simulink model "TESTENV_NAVI"  (R2020b)
settings: Solver=ode1  StartTime=tspan(1)  StopTime=tspan(2)  FixedStep=1/sensorFs.imuUpdateFs  RelTol=1e-3
values from neighbouring files (symbols this model uses):
  mag1 = double([Sensors.mag1.mag_x, Sensors.mag1.mag_y, Sensors.mag1.mag_z])    [navi_marg22.m]    (also in navi_marg24.m; navi_mvo17.m)
  mag2 = double([Sensors.mag2.mag_x, Sensors.mag2.mag_y, Sensors.mag2.mag_z])    [navi_marg22.m]    (also in navi_marg24.m; navi_mvo17.m)
undefined symbols (not defined in the file or in its folder): accel_x, accel_y, accel_z, ENUM_FlightTaskMode, flightControlMode, flightTaskMode, IMU1, IMU2, IMU3, mag_x, mag_y, mag_z, PlaneMode, SIM_SENSOR_SET, uavMode, VISLANDING_PARAM_V10, VISLANDING_PARAM_V1000
settings Model: PauseTimes=266.88  Creator=sl  LastModifiedBy=sl
settings SolverCC: AutoInsertRateTranBlk=on
settings OptimizationCC: DefaultParameterBehavior=Inlined  EnhancedBackFolding=on  PassReuseOutputArgsAs=Individual arguments  ZeroExternalMemoryAtStartup=off  ZeroInternalMemoryAtStartup=off  MaxStackSize=64  OptimizeBlockOrder=speed  DifferentSizesBufferReuse=on  OptimizationCustomize=off  EfficientTunableParamExpr=on
settings DebuggingCC: MultiTaskCondExecSysMsg=none  ParameterPrecisionLossMsg=none  ParameterTunabilityLossMsg=error  UnconnectedInputMsg=none  UnconnectedOutputMsg=none  UnconnectedLineMsg=none  BusObjectLabelMismatch=error
settings HardwareCC: ProdBitPerPointer=32  ProdBitPerSizeT=32  ProdBitPerPtrDiffT=32  ProdLargestAtomicInteger=Long  ProdLargestAtomicFloat=Double  ProdWordSize=32  ProdHWDeviceType=ARM Compatible->ARM Cortex
settings ModelReferenceCC: EnableParallelModelReferenceBuilds=on  ParallelModelReferenceMATLABWorkerInit=Load Top Model
settings SFSimCC: MATLABDynamicMemAlloc=off
settings RTWCC: Description=Embedded Coder  SystemTargetFile=ert.tlc  TemplateMakefile=ert_default_tmf  GenerateReport=on  Toolchain=GNU Tools for ARM Embedded Processors  IncludeHyperlinkInReport=on  LaunchReport=on  GenerateTraceInfo=on  GenerateTraceReport=on  GenerateTraceReportSl=on  GenerateTraceReportSf=on  GenerateTraceReportEml=on
settings CodeAppCC: ForceParamTrailComments=on  IgnoreCustomStorageClasses=off  OperatorAnnotations=on  SimulinkDataObjDesc=on  SFDataObjDesc=on  InsertBlockDesc=on
settings ERTTargetCC: InlinedParameterPlacement=NonHierarchical  ERTCustomFileTemplate=example_file_process.tlc

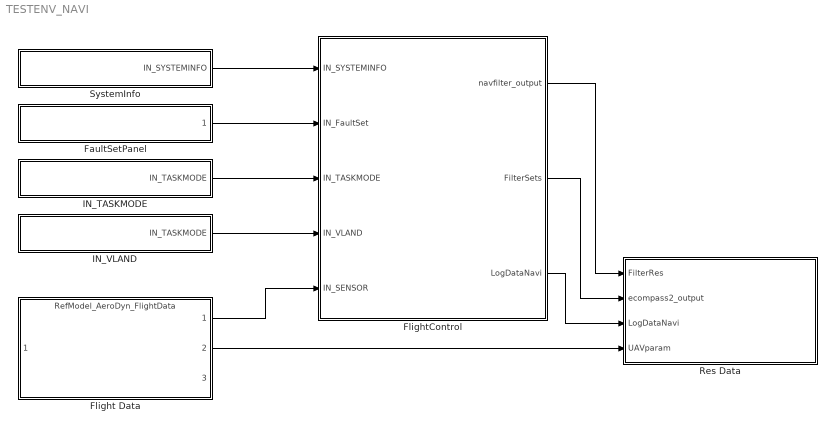
== system TESTENV_NAVI ==
  FaultSetPanel : ModelReference  ModelNameDialog=RefModel_FaultPanel  SimulationMode=Normal  ModelReferenceVersion=2.3
  Flight Data : ModelReference  DisableCoverage=on  ModelNameDialog=RefModel_AeroDyn_FlightData.slx  SimulationMode=Normal  ModelReferenceVersion=2.45
  FlightControl : Subsystem
  IN_TASKMODE : Subsystem
  IN_VLAND : Subsystem
  Res Data : Subsystem  VariantControl=SimulinkRunMode == 1
  SystemInfo : Subsystem
  wires:
  FlightControl/1(navfilter_output) -> Res Data/1(FilterRes)
  FlightControl/2(FilterSets) -> Res Data/2(ecompass2_output)
  Flight Data/1 -> FlightControl/5(IN_SENSOR)
  Flight Data/2 -> Res Data/4(UAVparam)
  FaultSetPanel/1 -> FlightControl/2(IN_FaultSet)
  SystemInfo/1(IN_SYSTEMINFO) -> FlightControl/1(IN_SYSTEMINFO)
  IN_TASKMODE/1(IN_TASKMODE) -> FlightControl/3(IN_TASKMODE)
  IN_VLAND/1(IN_TASKMODE) -> FlightControl/4(IN_VLAND)
  FlightControl/3(LogDataNavi) -> Res Data/3(LogDataNavi)

== system TESTENV_NAVI/FlightControl ==
  IN_SYSTEMINFO : Inport
  IN_FaultSet : Inport  Port=2
  IN_TASKMODE : Inport  Port=3
  IN_VLAND : Inport  Port=4
  IN_SENSOR : Inport  Port=5
  Bus Selector : BusSelector  OutputSignals=OUT_NaviFilter.Status.initialAlignmentComplete
  SensorAndNavigation1 : Subsystem
  TEST_Filter : Subsystem
  navfilter_output : Outport
  FilterSets : Outport  Port=2
  LogDataNavi : Outport  Port=3
  wires:
  SensorAndNavigation1/1(OUT_Navi) -> Bus Selector/1, navfilter_output/1
  IN_SENSOR/1 -> SensorAndNavigation1/1(IN_Sensor), TEST_Filter/1(In1)
  IN_FaultSet/1 -> SensorAndNavigation1/2(IN_FaultSet)
  TEST_Filter/1(Out1) -> FilterSets/1
  IN_SYSTEMINFO/1 -> SensorAndNavigation1/3(IN_SystemInfo)
  IN_TASKMODE/1 -> SensorAndNavigation1/4(IN_TASKMODE)
  IN_VLAND/1 -> SensorAndNavigation1/5(IN_VLandmark)
  SensorAndNavigation1/4(LogDataNavi) -> LogDataNavi/1

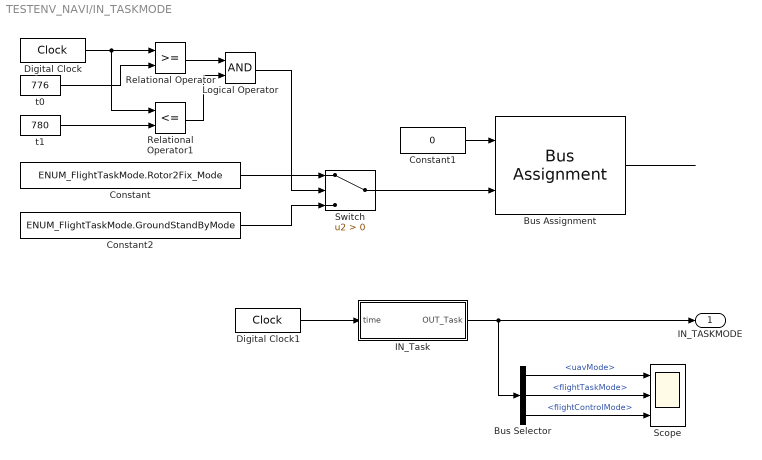
== system TESTENV_NAVI/IN_TASKMODE ==
  Bus Assignment : BusAssignment  AssignedSignals=flightTaskMode
  Bus Selector : BusSelector  OutputSignals=uavMode,flightTaskMode,flightControlMode
  Constant : Constant  Value=ENUM_FlightTaskMode.Rotor2Fix_Mode  OutDataTypeStr=Enum: ENUM_FlightTaskMode
  Constant1 : Constant  Value=0  OutDataTypeStr=Bus: BUS_TASK_PATH_OutParam
  Constant2 : Constant  Value=ENUM_FlightTaskMode.GroundStandByMode  OutDataTypeStr=Enum: ENUM_FlightTaskMode
  Digital Clock : DigitalClock  SampleTime=-1
  Digital Clock1 : DigitalClock  SampleTime=-1
  IN_Task : Subsystem
  Logical Operator : Logic  AllPortsSameDT=off  OutDataTypeStr=boolean
  Relational Operator : RelationalOperator  OutDataTypeStr=boolean  RndMeth=Simplest
  Relational Operator1 : RelationalOperator  Operator=<=  OutDataTypeStr=boolean  RndMeth=Simplest
  Scope : Scope  NumInputPorts=3
  Switch : Switch  Criteria=u2 > Threshold
  t0 : Constant  Value=776
  t1 : Constant  Value=780
  IN_TASKMODE : Outport
  wires:
  Bus Assignment/1 -> ?
  Constant/1 -> Switch/1
  Constant1/1 -> Bus Assignment/1
  Switch/1 -> Bus Assignment/2
  Constant2/1 -> Switch/3
  Logical Operator/1 -> Switch/2
  Digital Clock/1 -> Relational Operator1/1, Relational Operator/1
  t0/1 -> Relational Operator/2
  t1/1 -> Relational Operator1/2
  Relational Operator/1 -> Logical Operator/1
  Relational Operator1/1 -> Logical Operator/2
  Digital Clock1/1 -> IN_Task/1(time)
  IN_Task/1(OUT_Task) -> Bus Selector/1, IN_TASKMODE/1
  Bus Selector/1 -> Scope/1  "<uavMode>"
  Bus Selector/2 -> Scope/2  "<flightTaskMode>"
  Bus Selector/3 -> Scope/3  "<flightControlMode>"

== system TESTENV_NAVI/IN_VLAND ==
  Bus Assignment : BusAssignment  AssignedSignals=time
  Constant1 : Constant  Value=0  OutDataTypeStr=Bus: BUS_VISUALLANDING_INPUT
  IN_TASKMODE : Outport
  wires:
  Constant1/1 -> Bus Assignment/1
  Bus Assignment/1 -> IN_TASKMODE/1

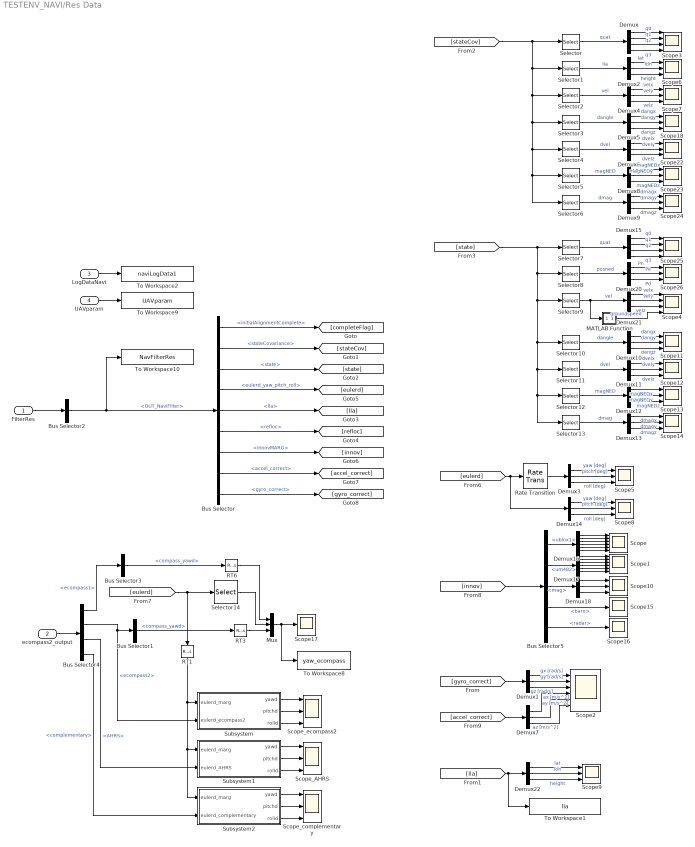
== system TESTENV_NAVI/Res Data ==
  FilterRes : Inport
  ecompass2_output : Inport  Port=2
  LogDataNavi : Inport  Port=3
  UAVparam : Inport  Port=4
  Bus Selector : BusSelector  OutputSignals=Status.initialAlignmentComplete,stateCovariance,state,eulerd_yaw_pitch_roll,lla,InitValue.refloc,innovMARG,accel_correct,gyro_correct
  Bus Selector1 : BusSelector  OutputSignals=compass_yawd
  Bus Selector2 : BusSelector  OutputSignals=OUT_NaviFilter
  Bus Selector3 : BusSelector  OutputSignals=compass_yawd
  Bus Selector4 : BusSelector  OutputSignals=ecompass1,ecompass2,AHRS,complementary
  Bus Selector5 : BusSelector  OutputSignals=ublox1,um482,mag,baro,radar
  Demux : Demux
  Demux{1..14,18,20..22} (18 alike) : Demux  Outputs=3
  Demux15 : Demux
  Demux16 : Demux  Outputs=6
  Demux17 : Demux  Outputs=6
  MATLAB Function : MATLAB Function  TreatAsAtomicUnit=on
  Mux : Mux  Inputs=3
  RT1 : RateTransition
  RT3 : RateTransition
  RT6 : RateTransition
  Rate Transition : RateTransition
  Scope : Scope  NumInputPorts=6
  Scope1 : Scope  NumInputPorts=6
  Scope{5..14,18,22..24,26} (15 alike) : Scope  NumInputPorts=3
  Scope15 : Scope
  Scope16 : Scope
  Scope17 : Scope
  Scope2 : Scope  NumInputPorts=6
  Scope25 : Scope  NumInputPorts=4
  Scope3 : Scope  NumInputPorts=4
  Scope4 : Scope  NumInputPorts=4
  Scope_AHRS : Scope  NumInputPorts=3
  Scope_complementary : Scope  NumInputPorts=3
  Scope_ecompass2 : Scope  NumInputPorts=3
  Selector : Selector  InputPortWidth=nStateMARG24  IndexOptions=Index vector (dialog)  Indices=[1:4]  OutputSizes=1
  Selector1 : Selector  InputPortWidth=nStateMARG24  IndexOptions=Index vector (dialog)  Indices=[5:7]  OutputSizes=1
  Selector10 : Selector  InputPortWidth=nStateMARG24  IndexOptions=Index vector (dialog)  Indices=[11:13]  OutputSizes=1
  Selector11 : Selector  InputPortWidth=nStateMARG24  IndexOptions=Index vector (dialog)  Indices=[14:16]  OutputSizes=1
  Selector12 : Selector  InputPortWidth=nStateMARG24  IndexOptions=Index vector (dialog)  Indices=[17:19]  OutputSizes=1
  Selector13 : Selector  InputPortWidth=nStateMARG24  IndexOptions=Index vector (dialog)  Indices=[20:22]  OutputSizes=1
  Selector14 : Selector  InputPortWidth=3  IndexOptions=Index vector (dialog)  Indices=1  OutputSizes=1
  Selector2 : Selector  InputPortWidth=nStateMARG24  IndexOptions=Index vector (dialog)  Indices=[8:10]  OutputSizes=1
  Selector3 : Selector  InputPortWidth=nStateMARG24  IndexOptions=Index vector (dialog)  Indices=[11:13]  OutputSizes=1
  Selector4 : Selector  InputPortWidth=nStateMARG24  IndexOptions=Index vector (dialog)  Indices=[14:16]  OutputSizes=1
  Selector5 : Selector  InputPortWidth=nStateMARG24  IndexOptions=Index vector (dialog)  Indices=[17:19]  OutputSizes=1
  Selector6 : Selector  InputPortWidth=nStateMARG24  IndexOptions=Index vector (dialog)  Indices=[20:22]  OutputSizes=1
  Selector7 : Selector  InputPortWidth=nStateMARG24  IndexOptions=Index vector (dialog)  Indices=[1:4]  OutputSizes=1
  Selector8 : Selector  InputPortWidth=nStateMARG24  IndexOptions=Index vector (dialog)  Indices=[5:7]  OutputSizes=1
  Selector9 : Selector  InputPortWidth=nStateMARG24  IndexOptions=Index vector (dialog)  Indices=[8:10]  OutputSizes=1
  Subsystem : Subsystem
  Subsystem1 : Subsystem
  Subsystem2 : Subsystem
  To Workspace1 : ToWorkspace  VariableName=lla  SaveFormat=Timeseries  SampleTime=-1
  To Workspace10 : ToWorkspace  VariableName=NavFilterRes  SaveFormat=Timeseries  SampleTime=-1
  To Workspace2 : ToWorkspace  VariableName=naviLogData1  SaveFormat=Timeseries  SampleTime=-1
  To Workspace8 : ToWorkspace  VariableName=yaw_ecompass  SaveFormat=Timeseries  SampleTime=-1
  To Workspace9 : ToWorkspace  VariableName=UAVparam  SaveFormat=Timeseries  SampleTime=-1
  wires:
  Demux13/1 -> Scope14/1  "dmagx"
  Demux21/3 -> Scope4/3  "velz"
  Demux12/1 -> Scope13/1  "magNEDx"
  Selector14/1 -> Mux/2
  Demux10/1 -> Scope11/1  "dangx"
  Demux12/2 -> Scope13/2  "magNEDy"
  Selector10/1 -> Demux10/1  "dangle"
  Demux15/4 -> Scope25/4  "q3"
  Selector1/1 -> Demux2/1  "lla"
  Demux3/2 -> Scope5/2  "pitch [deg]"
  [state] -> Selector8/1, Selector11/1, Selector12/1, Selector13/1, Selector10/1, Selector9/1, Selector7/1
  Demux5/2 -> Scope18/2  "dangy"
  Selector12/1 -> Demux12/1  "magNED"
  Selector13/1 -> Demux13/1  "dmag"
  Demux11/1 -> Scope12/1  "dvelx"
  [innov] -> Bus Selector5/1
  Demux11/2 -> Scope12/2  "dvely"
  Demux15/3 -> Scope25/3  "q2"
  Demux6/3 -> Scope22/3  "dvelz"
  Mux/1 -> To Workspace8/1, Scope17/1
  Demux15/2 -> Scope25/2  "q1"
  Bus Selector1/1 -> RT3/1  "<compass_yawd>"
  [eulerd] -> Demux14/1, Rate Transition/1
  [eulerd] -> Selector14/1, RT1/1
  Demux10/3 -> Scope11/3  "dangz"
  Demux21/1 -> Scope4/1  "velx"
  Demux/2 -> Scope3/2  "q1"
  Demux/1 -> Scope3/1  "q0"
  [stateCov] -> Selector/1, Selector3/1, Selector4/1, Selector5/1, Selector6/1, Selector2/1, Selector1/1
  Demux9/2 -> Scope24/2  "dmagy"
  Demux/3 -> Scope3/3  "q2"
  Selector2/1 -> Demux4/1  "vel"
  Demux13/2 -> Scope14/2  "dmagy"
  Selector6/1 -> Demux9/1  "dmag"
  RT3/1 -> Mux/3
  Demux/4 -> Scope3/4  "q3"
  Demux2/1 -> Scope6/1  "lat"
  Demux2/3 -> Scope6/3  "height"
  Selector/1 -> Demux/1  "quat"
  Demux5/3 -> Scope18/3  "dangz"
  Demux4/3 -> Scope7/3  "velz"
  Demux10/2 -> Scope11/2  "dangy"
  Demux4/2 -> Scope7/2  "vely"
  Demux8/2 -> Scope23/2  "magNEDy"
  Selector3/1 -> Demux5/1  "dangle"
  Demux2/2 -> Scope6/2  "lon"
  Selector5/1 -> Demux8/1  "magNED"
  Demux8/1 -> Scope23/1  "magNEDx"
  Demux6/2 -> Scope22/2  "dvely"
  Demux9/3 -> Scope24/3  "dmagz"
  Demux12/3 -> Scope13/3  "magNEDz"
  Demux3/3 -> Scope5/3  "roll [deg]"
  Demux21/2 -> Scope4/2  "vely"
  Demux8/3 -> Scope23/3  "magNEDz"
  Selector11/1 -> Demux11/1  "dvel"
  Selector9/1 -> MATLAB Function/1(vel), Demux21/1  "vel"
  Demux20/3 -> Scope26/3  "Pd"
  Selector7/1 -> Demux15/1  "quat"
  Demux13/3 -> Scope14/3  "dmagz"
  Demux20/2 -> Scope26/2  "Pe"
  Selector4/1 -> Demux6/1  "dvel"
  Selector8/1 -> Demux20/1  "posned"
  Demux3/1 -> Scope5/1  "yaw [deg]"
  Demux11/3 -> Scope12/3  "dvelz"
  Demux15/1 -> Scope25/1  "q0"
  Demux20/1 -> Scope26/1  "Pn"
  Demux5/1 -> Scope18/1  "dangx"
  Demux6/1 -> Scope22/1  "dvelx"
  Demux4/1 -> Scope7/1  "velx"
  Demux9/1 -> Scope24/1  "dmagx"
  FilterRes/1 -> Bus Selector2/1
  Bus Selector/4 -> [eulerd]  "<eulerd_yaw_pitch_roll>"
  Bus Selector/3 -> [state]  "<state>"
  Bus Selector/5 -> [lla]  "<lla>"
  Bus Selector/2 -> [stateCov]  "<stateCovariance>"
  Bus Selector/6 -> [refloc]  "<refloc>"
  Bus Selector/1 -> [completeFlag]  "<initialAlignmentComplete>"
  Bus Selector/7 -> [innov]  "<innovMARG>"
  ecompass2_output/1 -> Bus Selector4/1
  Bus Selector/8 -> [accel_correct]  "<accel_correct>"
  Bus Selector/9 -> [gyro_correct]  "<gyro_correct>"
  [gyro_correct] -> Demux1/1
  [accel_correct] -> Demux7/1
  Demux1/1 -> Scope2/1  "gx [rad/s]"
  Demux1/2 -> Scope2/2  "gy [rad/s]"
  Demux1/3 -> Scope2/3  "gz [rad/s]"
  Demux7/1 -> Scope2/4  "ax [m/s^2]"
  Demux7/2 -> Scope2/5  "ay [m/s^2]"
  Demux7/3 -> Scope2/6  "az [m/s^2]"
  UAVparam/1 -> To Workspace9/1
  Rate Transition/1 -> Demux3/1
  Demux14/1 -> Scope8/1  "yaw [deg]"
  Demux14/3 -> Scope8/3  "roll [deg]"
  Demux14/2 -> Scope8/2  "pitch [deg]"
  Demux22/2 -> Scope9/2  "lon"
  Demux22/3 -> Scope9/3  "height"
  Demux22/1 -> Scope9/1  "lat"
  [lla] -> To Workspace1/1, Demux22/1
  Bus Selector3/1 -> RT6/1  "<compass_yawd>"
  RT6/1 -> Mux/1
  Bus Selector4/2 -> Subsystem/2(eulerd_ecompass2), Bus Selector1/1  "<ecompass2>"
  Bus Selector4/1 -> Bus Selector3/1  "<ecompass1>"
  Bus Selector4/3 -> Subsystem1/2(eulerd_AHRS)  "<AHRS>"
  RT1/1 -> Subsystem2/1(eulerd_marg), Subsystem1/1(eulerd_marg), Subsystem/1(eulerd_marg)
  Subsystem/1(yawd) -> Scope_ecompass2/1
  Subsystem/2(pitchd) -> Scope_ecompass2/2
  Subsystem/3(rolld) -> Scope_ecompass2/3
  Subsystem1/3(rolld) -> Scope_AHRS/3
  Subsystem1/2(pitchd) -> Scope_AHRS/2
  Subsystem1/1(yawd) -> Scope_AHRS/1
  Subsystem2/1(yawd) -> Scope_complementary/1
  Subsystem2/2(pitchd) -> Scope_complementary/2
  Subsystem2/3(rolld) -> Scope_complementary/3
  Bus Selector4/4 -> Subsystem2/2(eulerd_complementary)  "<complementary>"
  MATLAB Function/1(y) -> Scope4/4  "groundspeed"
  Bus Selector2/1 -> To Workspace10/1, Bus Selector/1  "<OUT_NaviFilter>"
  LogDataNavi/1 -> To Workspace2/1
  Bus Selector5/1 -> Demux16/1  "<ublox1>"
  Demux16/1 -> Scope/1
  Demux16/2 -> Scope/2
  Demux16/3 -> Scope/3
  Demux16/4 -> Scope/4
  Demux16/5 -> Scope/5
  Demux16/6 -> Scope/6
  Demux17/6 -> Scope1/6
  Demux17/5 -> Scope1/5
  Demux17/4 -> Scope1/4
  Demux17/3 -> Scope1/3
  Demux17/2 -> Scope1/2
  Demux17/1 -> Scope1/1
  Bus Selector5/2 -> Demux17/1  "<um482>"
  Bus Selector5/3 -> Demux18/1  "<mag>"
  Demux18/1 -> Scope10/1
  Demux18/2 -> Scope10/2
  Demux18/3 -> Scope10/3
  Bus Selector5/4 -> Scope15/1  "<baro>"
  Bus Selector5/5 -> Scope16/1  "<radar>"

== system TESTENV_NAVI/SystemInfo ==
  Bus Assignment : BusAssignment  AssignedSignals=plane_model_control
  Constant : Constant  Value=PlaneMode.mode  OutDataTypeStr=Enum: ENUM_plane_mode
  Constant1 : Constant  Value=0  OutDataTypeStr=Bus: BUS_SYSTEMINFO_INPUT
  IN_SYSTEMINFO : Outport
  wires:
  Constant1/1 -> Bus Assignment/1
  Constant/1 -> Bus Assignment/2
  Bus Assignment/1 -> IN_SYSTEMINFO/1

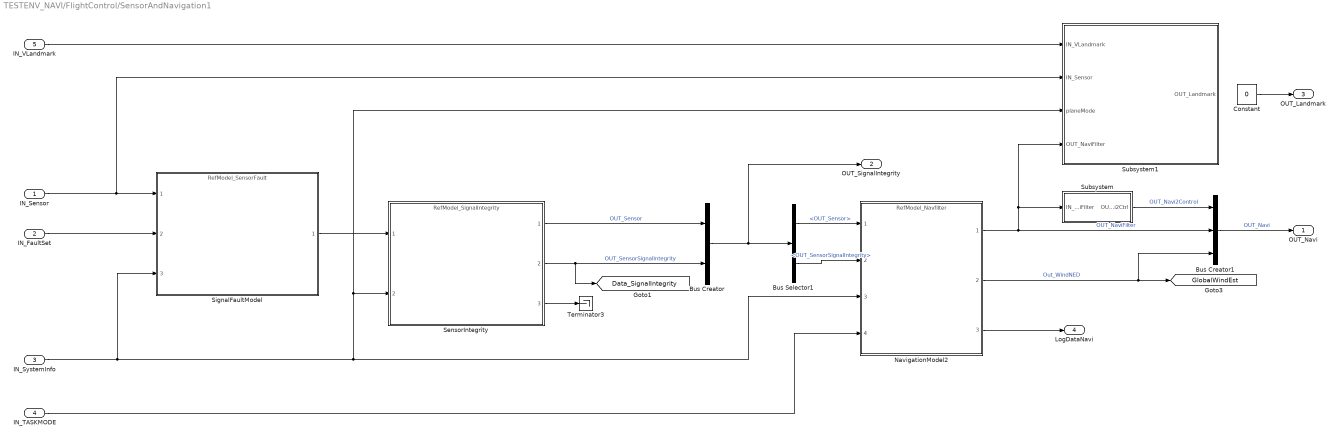
== system TESTENV_NAVI/FlightControl/SensorAndNavigation1 ==
  IN_Sensor : Inport
  IN_FaultSet : Inport  Port=2
  IN_SystemInfo : Inport  Port=3
  IN_TASKMODE : Inport  Port=4
  IN_VLandmark : Inport  Port=5
  Bus Creator : BusCreator  Inputs=2
  Bus Creator1 : BusCreator  Inputs=3
  Bus Selector1 : BusSelector  OutputSignals=OUT_Sensor,OUT_SensorSignalIntegrity
  Constant : Constant  Value=0  OutDataTypeStr=Bus: BUS_VISUALLANDING_LANDMARK
  NavigationModel2 : ModelReference  ModelNameDialog=RefModel_Navfilter  SimulationMode=Normal  CachedPortDiscreteRates=[0.004]  ModelReferenceVersion=2.1363
  SensorIntegrity : ModelReference  ModelNameDialog=RefModel_SignalIntegrity  SimulationMode=Normal  CachedPortDiscreteRates=[0.004]  ModelReferenceVersion=2.46
  SignalFaultModel : ModelReference  DisableCoverage=on  ModelNameDialog=RefModel_SensorFault.slx  SimulationMode=Normal  ModelReferenceVersion=2.1
  Subsystem : Subsystem
  Subsystem1 : Subsystem
  Terminator3 : Terminator
  OUT_Navi : Outport
  OUT_SignalIntegrity : Outport  Port=2
  OUT_Landmark : Outport  Port=3  OutDataTypeStr=Bus: BUS_VISUALLANDING_LANDMARK
  LogDataNavi : Outport  Port=4
  tag scope: Data_SignalIntegrity=global, GlobalWindEst=global
  wires:
  Bus Creator1/1 -> OUT_Navi/1  "OUT_Navi"
  IN_FaultSet/1 -> SignalFaultModel/2
  IN_Sensor/1 -> Subsystem1/2(IN_Sensor), SignalFaultModel/1
  SensorIntegrity/3 -> Terminator3/1
  SensorIntegrity/1 -> Bus Creator/1  "OUT_Sensor"
  SensorIntegrity/2 -> [Data_SignalIntegrity], Bus Creator/2  "OUT_SensorSignalIntegrity"
  SignalFaultModel/1 -> SensorIntegrity/1
  Subsystem/1(OUT_Navi2Ctrl) -> Bus Creator1/1  "OUT_Navi2Control"
  NavigationModel2/2 -> [GlobalWindEst], Bus Creator1/3  "Out_WindNED"
  Bus Creator/1 -> Bus Selector1/1, OUT_SignalIntegrity/1
  Bus Selector1/2 -> NavigationModel2/2  "<OUT_SensorSignalIntegrity>"
  Bus Selector1/1 -> NavigationModel2/1  "<OUT_Sensor>"
  NavigationModel2/1 -> Subsystem/1(IN_NaviFilter), Subsystem1/4(OUT_NaviFilter), Bus Creator1/2  "OUT_NaviFilter"
  IN_SystemInfo/1 -> Subsystem1/3(planeMode), SensorIntegrity/2, NavigationModel2/3, SignalFaultModel/3
  IN_TASKMODE/1 -> NavigationModel2/4
  IN_VLandmark/1 -> Subsystem1/1(IN_VLandmark)
  NavigationModel2/3 -> LogDataNavi/1
  Constant/1 -> OUT_Landmark/1

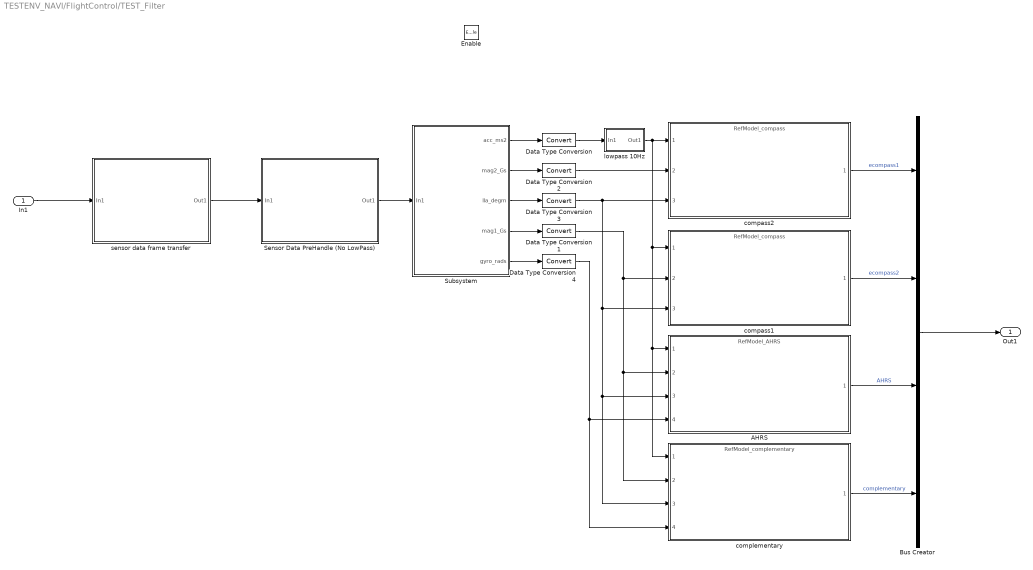
== system TESTENV_NAVI/FlightControl/TEST_Filter ==
  In1 : Inport
  Enable : EnablePort
  AHRS : ModelReference  ModelNameDialog=RefModel_AHRS.slx  SimulationMode=Normal  ModelReferenceVersion=2.3
  Bus Creator : BusCreator  Inputs=4
  Data Type Conversion{,1..4} (5 alike) : DataTypeConversion
  Sensor Data PreHandle (No LowPass) : Subsystem
  Subsystem : Subsystem
  compass1 : ModelReference  ModelNameDialog=RefModel_compass.slx  SimulationMode=Normal  ModelReferenceVersion=2.0
  compass2 : ModelReference  ModelNameDialog=RefModel_compass.slx  SimulationMode=Normal  ModelReferenceVersion=2.0
  complementary : ModelReference  ModelNameDialog=RefModel_complementary.slx  SimulationMode=Normal  ModelReferenceVersion=2.0
  lowpass 10Hz : Subsystem
  sensor data frame transfer : Subsystem
  Out1 : Outport
  wires:
  Sensor Data PreHandle (No LowPass)/1(Out1) -> Subsystem/1(In1)
  sensor data frame transfer/1(Out1) -> Sensor Data PreHandle (No LowPass)/1(In1)
  Data Type Conversion/1 -> lowpass 10Hz/1(In1)
  Subsystem/1(acc_ms2) -> Data Type Conversion/1
  Subsystem/2(mag2_Gs) -> Data Type Conversion2/1
  Data Type Conversion2/1 -> compass2/2
  lowpass 10Hz/1(Out1) -> complementary/1, AHRS/1, compass1/1, compass2/1
  Subsystem/4(mag1_Gs) -> Data Type Conversion1/1
  Data Type Conversion4/1 -> complementary/4, AHRS/4
  Data Type Conversion3/1 -> complementary/3, AHRS/3, compass1/3, compass2/3
  Data Type Conversion1/1 -> complementary/2, AHRS/2, compass1/2
  Subsystem/3(lla_degm) -> Data Type Conversion3/1
  Subsystem/5(gyro_rads) -> Data Type Conversion4/1
  AHRS/1 -> Bus Creator/3  "AHRS"
  complementary/1 -> Bus Creator/4  "complementary"
  Bus Creator/1 -> Out1/1
  compass2/1 -> Bus Creator/1  "ecompass1"
  compass1/1 -> Bus Creator/2  "ecompass2"
  In1/1 -> sensor data frame transfer/1(In1)

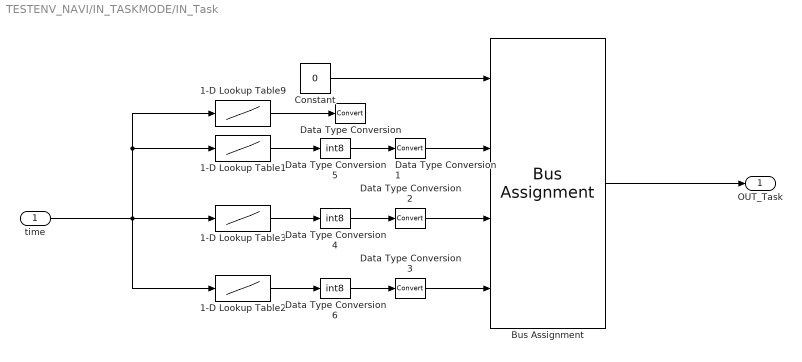
== system TESTENV_NAVI/IN_TASKMODE/IN_Task ==
  time : Inport
  1-D Lookup Table1 : Lookup_n-D  NumberOfTableDimensions=1  BreakpointsForDimension1=IN_Task.time_cal(1:end-20)  Table=IN_Task.uavMode(1:end-20)  InterpMethod=Flat  ExtrapMethod=Clip  InternalRulePriority=Speed  RndMeth=Simplest  InputSameDT=on
  1-D Lookup Table2 : Lookup_n-D  NumberOfTableDimensions=1  BreakpointsForDimension1=IN_Task.time_cal(1:end-20)  Table=IN_Task.flightControlMode(1:end-20)  InterpMethod=Flat  ExtrapMethod=Clip  InternalRulePriority=Speed  RndMeth=Simplest  InputSameDT=on
  1-D Lookup Table3 : Lookup_n-D  NumberOfTableDimensions=1  BreakpointsForDimension1=IN_Task.time_cal(1:end-20)  Table=IN_Task.flightTaskMode(1:end-20)  InterpMethod=Flat  ExtrapMethod=Clip  InternalRulePriority=Speed  RndMeth=Simplest  InputSameDT=on
  1-D Lookup Table9 : Lookup_n-D  NumberOfTableDimensions=1  BreakpointsForDimension1=IN_Task.time_cal(1:end-20)  Table=IN_Task.time_cal(1:end-20)  InterpMethod=Flat  ExtrapMethod=Clip  InternalRulePriority=Speed  RndMeth=Simplest  InputSameDT=on
  Bus Assignment : BusAssignment  AssignedSignals=uavMode,flightTaskMode,flightControlMode
  Constant : Constant  Value=0  OutDataTypeStr=Bus: BUS_TASK_PATH_OutParam
  Data Type Conversion{,1..3} (4 alike) : DataTypeConversion
  Data Type Conversion4 : DataTypeConversion  OutDataTypeStr=int8
  Data Type Conversion5 : DataTypeConversion  OutDataTypeStr=int8
  Data Type Conversion6 : DataTypeConversion  OutDataTypeStr=int8
  OUT_Task : Outport
  wires:
  Bus Assignment/1 -> OUT_Task/1
  1-D Lookup Table9/1 -> Data Type Conversion/1
  1-D Lookup Table1/1 -> Data Type Conversion5/1
  1-D Lookup Table3/1 -> Data Type Conversion4/1
  1-D Lookup Table2/1 -> Data Type Conversion6/1
  time/1 -> 1-D Lookup Table2/1, 1-D Lookup Table3/1, 1-D Lookup Table1/1, 1-D Lookup Table9/1
  Constant/1 -> Bus Assignment/1
  Data Type Conversion1/1 -> Bus Assignment/2
  Data Type Conversion2/1 -> Bus Assignment/3
  Data Type Conversion3/1 -> Bus Assignment/4
  Data Type Conversion6/1 -> Data Type Conversion3/1
  Data Type Conversion5/1 -> Data Type Conversion1/1
  Data Type Conversion4/1 -> Data Type Conversion2/1

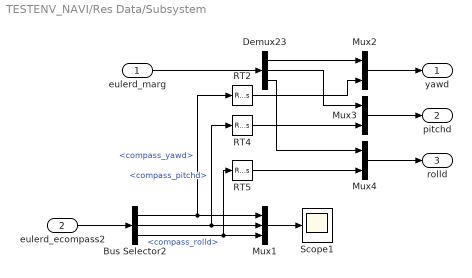
== system TESTENV_NAVI/Res Data/Subsystem ==
  eulerd_marg : Inport
  eulerd_ecompass2 : Inport  Port=2
  Bus Selector2 : BusSelector  OutputSignals=compass_yawd,compass_pitchd,compass_rolld
  Demux23 : Demux  Outputs=3
  Mux1 : Mux  Inputs=3
  Mux2 : Mux  Inputs=2
  Mux3 : Mux  Inputs=2
  Mux4 : Mux  Inputs=2
  RT2 : RateTransition
  RT4 : RateTransition
  RT5 : RateTransition
  Scope1 : Scope
  yawd : Outport
  pitchd : Outport  Port=2
  rolld : Outport  Port=3
  wires:
  RT4/1 -> Mux3/2
  Demux23/1 -> Mux2/1
  RT2/1 -> Mux2/2
  Mux1/1 -> Scope1/1
  Bus Selector2/2 -> RT4/1, Mux1/2  "<compass_pitchd>"
  Demux23/3 -> Mux4/1
  eulerd_marg/1 -> Demux23/1
  Bus Selector2/3 -> RT5/1, Mux1/3  "<compass_rolld>"
  RT5/1 -> Mux4/2
  Demux23/2 -> Mux3/1
  Bus Selector2/1 -> Mux1/1, RT2/1  "<compass_yawd>"
  Mux4/1 -> rolld/1
  eulerd_ecompass2/1 -> Bus Selector2/1
  Mux3/1 -> pitchd/1
  Mux2/1 -> yawd/1

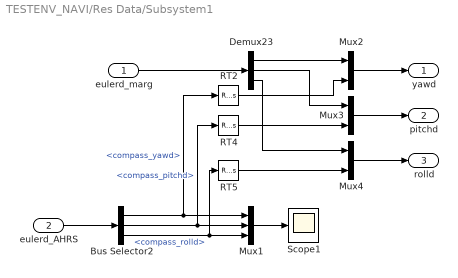
== system TESTENV_NAVI/Res Data/Subsystem1 ==
  eulerd_marg : Inport
  eulerd_AHRS : Inport  Port=2
  Bus Selector2 : BusSelector  OutputSignals=compass_yawd,compass_pitchd,compass_rolld
  Demux23 : Demux  Outputs=3
  Mux1 : Mux  Inputs=3
  Mux2 : Mux  Inputs=2
  Mux3 : Mux  Inputs=2
  Mux4 : Mux  Inputs=2
  RT2 : RateTransition
  RT4 : RateTransition
  RT5 : RateTransition
  Scope1 : Scope
  yawd : Outport
  pitchd : Outport  Port=2
  rolld : Outport  Port=3
  wires:
  Mux2/1 -> yawd/1
  Mux3/1 -> pitchd/1
  eulerd_AHRS/1 -> Bus Selector2/1
  Mux4/1 -> rolld/1
  Bus Selector2/1 -> RT2/1, Mux1/1  "<compass_yawd>"
  Demux23/2 -> Mux3/1
  RT5/1 -> Mux4/2
  Bus Selector2/3 -> Mux1/3, RT5/1  "<compass_rolld>"
  eulerd_marg/1 -> Demux23/1
  Demux23/3 -> Mux4/1
  Bus Selector2/2 -> Mux1/2, RT4/1  "<compass_pitchd>"
  Mux1/1 -> Scope1/1
  RT2/1 -> Mux2/2
  Demux23/1 -> Mux2/1
  RT4/1 -> Mux3/2

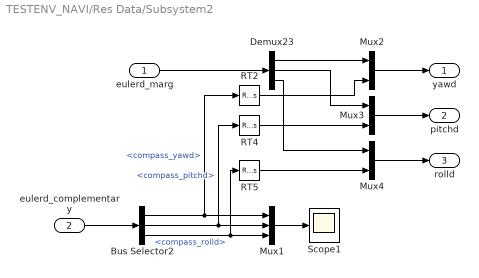
== system TESTENV_NAVI/Res Data/Subsystem2 ==
  eulerd_marg : Inport
  eulerd_complementary : Inport  Port=2
  Bus Selector2 : BusSelector  OutputSignals=compass_yawd,compass_pitchd,compass_rolld
  Demux23 : Demux  Outputs=3
  Mux1 : Mux  Inputs=3
  Mux2 : Mux  Inputs=2
  Mux3 : Mux  Inputs=2
  Mux4 : Mux  Inputs=2
  RT2 : RateTransition
  RT4 : RateTransition
  RT5 : RateTransition
  Scope1 : Scope
  yawd : Outport
  pitchd : Outport  Port=2
  rolld : Outport  Port=3
  wires:
  RT4/1 -> Mux3/2
  Demux23/1 -> Mux2/1
  RT2/1 -> Mux2/2
  Mux1/1 -> Scope1/1
  Bus Selector2/2 -> RT4/1, Mux1/2  "<compass_pitchd>"
  Demux23/3 -> Mux4/1
  eulerd_marg/1 -> Demux23/1
  Bus Selector2/3 -> RT5/1, Mux1/3  "<compass_rolld>"
  RT5/1 -> Mux4/2
  Demux23/2 -> Mux3/1
  Bus Selector2/1 -> Mux1/1, RT2/1  "<compass_yawd>"
  Mux4/1 -> rolld/1
  eulerd_complementary/1 -> Bus Selector2/1
  Mux3/1 -> pitchd/1
  Mux2/1 -> yawd/1

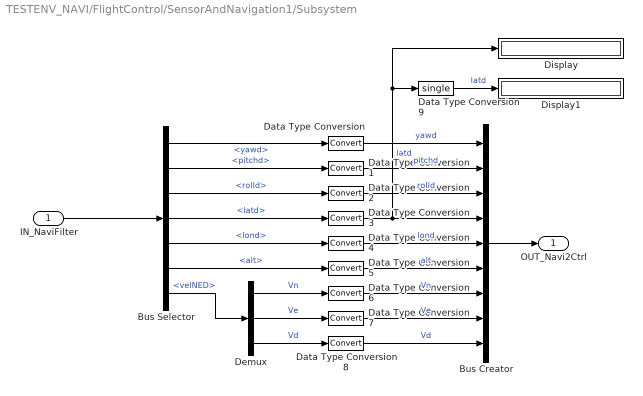
== system TESTENV_NAVI/FlightControl/SensorAndNavigation1/Subsystem ==
  IN_NaviFilter : Inport
  Bus Creator : BusCreator  Inputs=9
  Bus Selector : BusSelector  OutputSignals=yawd,pitchd,rolld,latd,lond,alt,velNED
  Data Type Conversion{,1..8} (9 alike) : DataTypeConversion
  Data Type Conversion9 : DataTypeConversion  OutDataTypeStr=single
  Demux : Demux  Outputs=3
  Display : Display
  Display1 : Display
  OUT_Navi2Ctrl : Outport
  wires:
  IN_NaviFilter/1 -> Bus Selector/1
  Bus Selector/7 -> Demux/1  "<velNED>"
  Bus Selector/1 -> Data Type Conversion/1  "<yawd>"
  Bus Selector/2 -> Data Type Conversion1/1  "<pitchd>"
  Bus Selector/3 -> Data Type Conversion2/1  "<rolld>"
  Bus Selector/4 -> Data Type Conversion3/1  "<latd>"
  Bus Selector/5 -> Data Type Conversion4/1  "<lond>"
  Bus Selector/6 -> Data Type Conversion5/1  "<alt>"
  Demux/3 -> Data Type Conversion8/1  "Vd"
  Demux/2 -> Data Type Conversion7/1  "Ve"
  Demux/1 -> Data Type Conversion6/1  "Vn"
  Bus Creator/1 -> OUT_Navi2Ctrl/1
  Data Type Conversion/1 -> Bus Creator/1  "yawd"
  Data Type Conversion1/1 -> Bus Creator/2  "pitchd"
  Data Type Conversion2/1 -> Bus Creator/3  "rolld"
  Data Type Conversion3/1 -> Data Type Conversion9/1, Display/1, Bus Creator/4  "latd"
  Data Type Conversion4/1 -> Bus Creator/5  "lond"
  Data Type Conversion6/1 -> Bus Creator/7  "Vn"
  Data Type Conversion5/1 -> Bus Creator/6  "alt"
  Data Type Conversion7/1 -> Bus Creator/8  "Ve"
  Data Type Conversion8/1 -> Bus Creator/9  "Vd"
  Data Type Conversion9/1 -> Display1/1  "latd"

== system TESTENV_NAVI/FlightControl/SensorAndNavigation1/Subsystem1 ==
  IN_VLandmark : Inport
  IN_Sensor : Inport  Port=2
  planeMode : Inport  Port=3
  OUT_NaviFilter : Inport  Port=4
  Bus Selector : BusSelector  OutputSignals=plane_model_control
  Bus Selector1 : BusSelector  OutputSignals=enableCompileInSystem
  Constant : Constant  Value=VISLANDING_PARAM_V1000  OutDataTypeStr=Bus: BUS_VISUALLANDING_PARAM
  Constant2 : Constant  Value=VISLANDING_PARAM_V10  OutDataTypeStr=Bus: BUS_VISUALLANDING_PARAM
  Select VisLandParam : MATLAB Function  TreatAsAtomicUnit=on
  Subsystem : Subsystem  Commented=on
  OUT_Landmark : Outport
  wires:
  IN_VLandmark/1 -> Subsystem/1(IN_VLAND)
  IN_Sensor/1 -> Subsystem/2(IN_SENSOR)
  OUT_NaviFilter/1 -> Subsystem/3(OUT_NAVI2FIRM)
  planeMode/1 -> Bus Selector/1, Subsystem/4(planeMode)
  Subsystem/1(OUT_LANDMARK) -> OUT_Landmark/1
  Constant/1 -> Select VisLandParam/2(P_V1000)
  Constant2/1 -> Select VisLandParam/3(P_V10)
  Bus Selector/1 -> Select VisLandParam/1(planeMode)  "<plane_model_control>"
  Select VisLandParam/1(P) -> Bus Selector1/1
  Bus Selector1/1 -> Subsystem/Enable  "<enableCompileInSystem>"

== system TESTENV_NAVI/FlightControl/TEST_Filter/Sensor Data PreHandle (No LowPass) ==
  In1 : Inport
  Bus Assignment : BusAssignment  AssignedSignals=IMU1,IMU2,IMU3,mag1,mag2
  Bus Selector : BusSelector  OutputSignals=IMU1,IMU2,IMU3
  Bus Selector1 : BusSelector  OutputSignals=mag1,mag2
  Subsystem : Subsystem
  Subsystem1 : Subsystem
  Subsystem2 : Subsystem
  Subsystem3 : Subsystem
  Subsystem4 : Subsystem
  Out1 : Outport
  wires:
  Bus Selector1/2 -> Subsystem4/1(In1)  "<mag2>"
  Bus Selector1/1 -> Subsystem3/1(In1)  "<mag1>"
  Bus Selector/3 -> Subsystem2/1(In1)  "<IMU3>"
  Bus Selector/2 -> Subsystem1/1(In1)  "<IMU2>"
  Bus Selector/1 -> Subsystem/1(In1)  "<IMU1>"
  Subsystem4/1(Out1) -> Bus Assignment/6  "mag2"
  Subsystem3/1(Out1) -> Bus Assignment/5  "mag1"
  In1/1 -> Bus Selector/1, Bus Assignment/1, Bus Selector1/1
  Bus Assignment/1 -> Out1/1
  Subsystem2/1(Out1) -> Bus Assignment/4  "IMU3"
  Subsystem1/1(Out1) -> Bus Assignment/3  "IMU2"
  Subsystem/1(Out1) -> Bus Assignment/2  "IMU1"

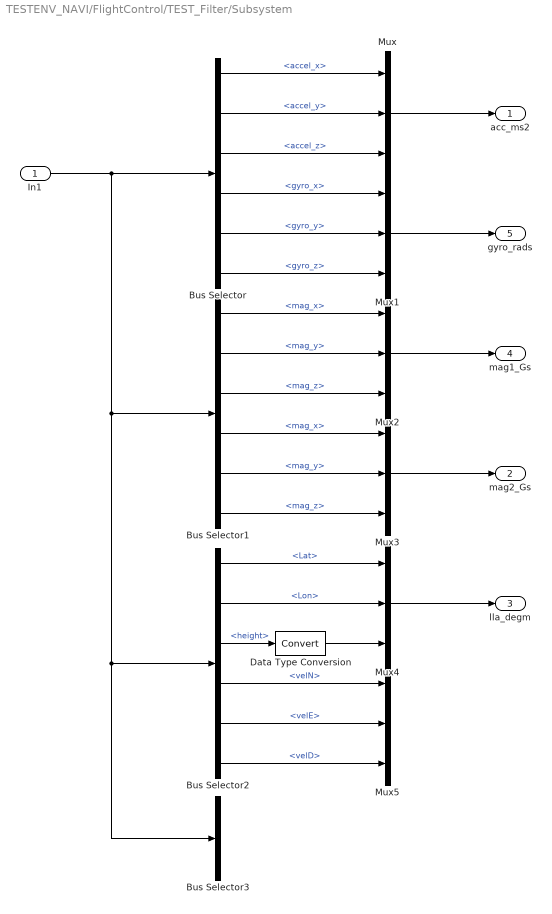
== system TESTENV_NAVI/FlightControl/TEST_Filter/Subsystem ==
  In1 : Inport
  Bus Selector : BusSelector  OutputSignals=IMU1.accel_x,IMU1.accel_y,IMU1.accel_z,IMU1.gyro_x,IMU1.gyro_y,IMU1.gyro_z
  Bus Selector1 : BusSelector  OutputSignals=mag1.mag_x,mag1.mag_y,mag1.mag_z,mag2.mag_x,mag2.mag_y,mag2.mag_z
  Bus Selector2 : BusSelector  OutputSignals=ublox1.Lat,ublox1.Lon,ublox1.height,ublox1.velN,ublox1.velE,ublox1.velD
  Bus Selector3 : BusSelector  OutputSignals=baro1.alt_baro,radar1.Range
  Data Type Conversion : DataTypeConversion
  Mux{,1..5} (6 alike) : Mux  Inputs=3
  acc_ms2 : Outport
  mag2_Gs : Outport  Port=2
  lla_degm : Outport  Port=3
  mag1_Gs : Outport  Port=4
  gyro_rads : Outport  Port=5
  wires:
  In1/1 -> Bus Selector3/1, Bus Selector2/1, Bus Selector1/1, Bus Selector/1
  Bus Selector/1 -> Mux/1  "<accel_x>"
  Bus Selector/2 -> Mux/2  "<accel_y>"
  Bus Selector/3 -> Mux/3  "<accel_z>"
  Bus Selector/4 -> Mux1/1  "<gyro_x>"
  Bus Selector/5 -> Mux1/2  "<gyro_y>"
  Bus Selector/6 -> Mux1/3  "<gyro_z>"
  Mux/1 -> acc_ms2/1
  Bus Selector1/1 -> Mux2/1  "<mag_x>"
  Bus Selector1/2 -> Mux2/2  "<mag_y>"
  Bus Selector1/3 -> Mux2/3  "<mag_z>"
  Bus Selector1/4 -> Mux3/1  "<mag_x>"
  Bus Selector1/5 -> Mux3/2  "<mag_y>"
  Bus Selector1/6 -> Mux3/3  "<mag_z>"
  Bus Selector2/6 -> Mux5/3  "<velD>"
  Bus Selector2/5 -> Mux5/2  "<velE>"
  Bus Selector2/4 -> Mux5/1  "<velN>"
  Bus Selector2/3 -> Data Type Conversion/1  "<height>"
  Bus Selector2/2 -> Mux4/2  "<Lon>"
  Bus Selector2/1 -> Mux4/1  "<Lat>"
  Mux4/1 -> lla_degm/1
  Data Type Conversion/1 -> Mux4/3
  Mux3/1 -> mag2_Gs/1
  Mux2/1 -> mag1_Gs/1
  Mux1/1 -> gyro_rads/1

== system TESTENV_NAVI/FlightControl/TEST_Filter/lowpass 10Hz ==
  In1 : Inport
  Demux : Demux  Outputs=3
  Mux : Mux  Inputs=3
  Mux1 : Mux  Inputs=2
  Mux2 : Mux  Inputs=2
  Mux3 : Mux  Inputs=2
  Scope : Scope  NumInputPorts=3
  Transfer Fcn : TransferFcn  Denominator=[.1 1]
  Transfer Fcn1 : TransferFcn  Denominator=[.1 1]
  Transfer Fcn2 : TransferFcn  Denominator=[.1 1]
  Out1 : Outport
  wires:
  In1/1 -> Demux/1
  Demux/1 -> Mux1/1, Transfer Fcn/1  "orignial x"
  Demux/2 -> Mux2/1, Transfer Fcn1/1  "orignial y"
  Mux/1 -> Out1/1
  Transfer Fcn1/1 -> Mux2/2, Mux/2  "filter y"
  Transfer Fcn2/1 -> Mux3/2, Mux/3  "filter z"
  Transfer Fcn/1 -> Mux1/2, Mux/1  "filter x"
  Demux/3 -> Mux3/1, Transfer Fcn2/1  "orignial z"
  Mux1/1 -> Scope/1  "ax"
  Mux2/1 -> Scope/2  "ay"
  Mux3/1 -> Scope/3  "az"

== system TESTENV_NAVI/FlightControl/TEST_Filter/sensor data frame transfer ==
  In1 : Inport
  Bus Assignment : BusAssignment  AssignedSignals=IMU1,IMU2,IMU3,mag1,mag2
  Bus Selector : BusSelector  OutputSignals=IMU1,IMU2,IMU3
  Bus Selector1 : BusSelector  OutputSignals=mag1,mag2
  SensorFrame to BodyFrame : Subsystem
  SensorFrame to BodyFrame1 : Subsystem
  SensorFrame to BodyFrame2 : Subsystem
  SensorFrame to BodyFrame3 : Subsystem
  SensorFrame to BodyFrame4 : Subsystem
  Out1 : Outport
  wires:
  Bus Selector/1 -> SensorFrame to BodyFrame/1(In1)  "<IMU1>"
  Bus Selector/2 -> SensorFrame to BodyFrame1/1(In1)  "<IMU2>"
  Bus Selector/3 -> SensorFrame to BodyFrame2/1(In1)  "<IMU3>"
  SensorFrame to BodyFrame/1(Out1) -> Bus Assignment/2  "IMU1"
  SensorFrame to BodyFrame1/1(Out1) -> Bus Assignment/3  "IMU2"
  SensorFrame to BodyFrame2/1(Out1) -> Bus Assignment/4  "IMU3"
  Bus Assignment/1 -> Out1/1
  In1/1 -> Bus Selector1/1, Bus Assignment/1, Bus Selector/1
  Bus Selector1/1 -> SensorFrame to BodyFrame3/1(In1)  "<mag1>"
  Bus Selector1/2 -> SensorFrame to BodyFrame4/1(In1)  "<mag2>"
  SensorFrame to BodyFrame3/1(Out1) -> Bus Assignment/5  "mag1"
  SensorFrame to BodyFrame4/1(Out1) -> Bus Assignment/6  "mag2"

== system TESTENV_NAVI/FlightControl/SensorAndNavigation1/Subsystem1/Subsystem ==
  IN_VLAND : Inport
  IN_SENSOR : Inport  Port=2
  OUT_NAVI2FIRM : Inport  Port=3
  planeMode : Inport  Port=4
  Enable : EnablePort
  SubModel_VisualLanding : ModelReference  ModelNameDialog=RefModel_VisualLanding.slx  SimulationMode=Normal  ModelReferenceVersion=2.203
  OUT_LANDMARK : Outport
  wires:
  planeMode/1 -> SubModel_VisualLanding/3
  IN_VLAND/1 -> SubModel_VisualLanding/1
  SubModel_VisualLanding/1 -> OUT_LANDMARK/1
  IN_SENSOR/1 -> SubModel_VisualLanding/2
  OUT_NAVI2FIRM/1 -> SubModel_VisualLanding/4

== system TESTENV_NAVI/FlightControl/TEST_Filter/Sensor Data PreHandle (No LowPass)/Subsystem ==
  In1 : Inport
  Bus Assignment : BusAssignment  AssignedSignals=accel_x,accel_y,accel_z
  Bus Selector1 : BusSelector  OutputSignals=accel_x,accel_y,accel_z
  Gain10 : Gain  Gain=-1
  Gain11 : Gain  Gain=-1
  Gain9 : Gain  Gain=-1
  Out1 : Outport
  wires:
  Bus Selector1/3 -> Gain11/1  "<accel_z>"
  In1/1 -> Bus Assignment/1, Bus Selector1/1
  Bus Selector1/2 -> Gain10/1  "<accel_y>"
  Bus Selector1/1 -> Gain9/1  "<accel_x>"
  Gain9/1 -> Bus Assignment/2  "ax"
  Gain10/1 -> Bus Assignment/3  "ay"
  Gain11/1 -> Bus Assignment/4  "az"
  Bus Assignment/1 -> Out1/1

== system TESTENV_NAVI/FlightControl/TEST_Filter/Sensor Data PreHandle (No LowPass)/Subsystem1 ==
  In1 : Inport
  Bus Assignment : BusAssignment  AssignedSignals=accel_x,accel_y,accel_z
  Bus Selector1 : BusSelector  OutputSignals=accel_x,accel_y,accel_z
  Gain10 : Gain  Gain=-1
  Gain11 : Gain  Gain=-1
  Gain9 : Gain  Gain=-1
  Out1 : Outport
  wires:
  Bus Assignment/1 -> Out1/1
  Gain11/1 -> Bus Assignment/4  "az"
  Gain10/1 -> Bus Assignment/3  "ay"
  Gain9/1 -> Bus Assignment/2  "ax"
  Bus Selector1/1 -> Gain9/1  "<accel_x>"
  Bus Selector1/2 -> Gain10/1  "<accel_y>"
  In1/1 -> Bus Selector1/1, Bus Assignment/1
  Bus Selector1/3 -> Gain11/1  "<accel_z>"

== system TESTENV_NAVI/FlightControl/TEST_Filter/Sensor Data PreHandle (No LowPass)/Subsystem2 ==
  In1 : Inport
  Bus Assignment : BusAssignment  AssignedSignals=accel_x,accel_y,accel_z
  Bus Selector1 : BusSelector  OutputSignals=accel_x,accel_y,accel_z
  Gain10 : Gain  Gain=-1
  Gain11 : Gain  Gain=-1
  Gain9 : Gain  Gain=-1
  Out1 : Outport
  wires:
  Bus Selector1/3 -> Gain11/1  "<accel_z>"
  In1/1 -> Bus Assignment/1, Bus Selector1/1
  Bus Selector1/2 -> Gain10/1  "<accel_y>"
  Bus Selector1/1 -> Gain9/1  "<accel_x>"
  Gain9/1 -> Bus Assignment/2  "ax"
  Gain10/1 -> Bus Assignment/3  "ay"
  Gain11/1 -> Bus Assignment/4  "az"
  Bus Assignment/1 -> Out1/1

== system TESTENV_NAVI/FlightControl/TEST_Filter/Sensor Data PreHandle (No LowPass)/Subsystem3 ==
  In1 : Inport
  Bus Assignment : BusAssignment  AssignedSignals=mag_x,mag_y,mag_z
  Bus Selector : BusSelector  OutputSignals=mag_x,mag_y,mag_z
  Gs to uT1 : Gain  Gain=100
  Gs to uT2 : Gain  Gain=100
  Gs to uT3 : Gain  Gain=100
  Out1 : Outport
  wires:
  Bus Selector/3 -> Gs to uT3/1  "<mag_z>"
  Bus Selector/2 -> Gs to uT2/1  "<mag_y>"
  Bus Selector/1 -> Gs to uT1/1  "<mag_x>"
  In1/1 -> Bus Assignment/1, Bus Selector/1
  Gs to uT1/1 -> Bus Assignment/2  "mag_x"
  Gs to uT2/1 -> Bus Assignment/3  "mag_y"
  Gs to uT3/1 -> Bus Assignment/4  "mag_z"
  Bus Assignment/1 -> Out1/1

== system TESTENV_NAVI/FlightControl/TEST_Filter/Sensor Data PreHandle (No LowPass)/Subsystem4 ==
  In1 : Inport
  Bus Assignment : BusAssignment  AssignedSignals=mag_x,mag_y,mag_z
  Bus Selector : BusSelector  OutputSignals=mag_x,mag_y,mag_z
  Gs to uT1 : Gain  Gain=100
  Gs to uT2 : Gain  Gain=100
  Gs to uT3 : Gain  Gain=100
  Out1 : Outport
  wires:
  Bus Assignment/1 -> Out1/1
  Gs to uT3/1 -> Bus Assignment/4  "mag_z"
  Gs to uT2/1 -> Bus Assignment/3  "mag_y"
  Gs to uT1/1 -> Bus Assignment/2  "mag_x"
  In1/1 -> Bus Selector/1, Bus Assignment/1
  Bus Selector/1 -> Gs to uT1/1  "<mag_x>"
  Bus Selector/2 -> Gs to uT2/1  "<mag_y>"
  Bus Selector/3 -> Gs to uT3/1  "<mag_z>"

== system TESTENV_NAVI/FlightControl/TEST_Filter/sensor data frame transfer/SensorFrame to BodyFrame ==
  In1 : Inport
  Bus Creator : BusCreator  Inputs=8
  Bus Selector : BusSelector  OutputSignals=time,accel_x,accel_y,accel_z,gyro_x,gyro_y,gyro_z,nChange
  Frame Transfer : Subsystem
  Frame Transfer1 : Subsystem
  Out1 : Outport
  wires:
  Bus Selector/1 -> Bus Creator/1  "<time>"
  Bus Creator/1 -> Out1/1
  In1/1 -> Bus Selector/1
  Bus Selector/2 -> Frame Transfer/1(In1)  "<accel_x>"
  Bus Selector/3 -> Frame Transfer/2(In2)  "<accel_y>"
  Bus Selector/4 -> Frame Transfer/3(In3)  "<accel_z>"
  Frame Transfer/1(Out1) -> Bus Creator/2  "accel_x"
  Frame Transfer/2(Out2) -> Bus Creator/3  "accel_y"
  Frame Transfer/3(Out3) -> Bus Creator/4  "accel_z"
  Bus Selector/5 -> Frame Transfer1/1(In1)  "<gyro_x>"
  Bus Selector/6 -> Frame Transfer1/2(In2)  "<gyro_y>"
  Bus Selector/7 -> Frame Transfer1/3(In3)  "<gyro_z>"
  Frame Transfer1/1(Out1) -> Bus Creator/5  "gyro_x"
  Frame Transfer1/2(Out2) -> Bus Creator/6  "gyro_y"
  Frame Transfer1/3(Out3) -> Bus Creator/7  "gyro_z"
  Bus Selector/8 -> Bus Creator/8  "<nChange>"

== system TESTENV_NAVI/FlightControl/TEST_Filter/sensor data frame transfer/SensorFrame to BodyFrame1 ==
  In1 : Inport
  Bus Creator : BusCreator  Inputs=8
  Bus Selector : BusSelector  OutputSignals=time,accel_x,accel_y,accel_z,gyro_x,gyro_y,gyro_z,nChange
  Frame Transfer : Subsystem
  Frame Transfer1 : Subsystem
  Out1 : Outport
  wires:
  Frame Transfer1/3(Out3) -> Bus Creator/7  "gyro_z"
  Frame Transfer1/2(Out2) -> Bus Creator/6  "gyro_y"
  Frame Transfer1/1(Out1) -> Bus Creator/5  "gyro_x"
  Bus Selector/7 -> Frame Transfer1/3(In3)  "<gyro_z>"
  Bus Selector/6 -> Frame Transfer1/2(In2)  "<gyro_y>"
  Bus Selector/5 -> Frame Transfer1/1(In1)  "<gyro_x>"
  Frame Transfer/3(Out3) -> Bus Creator/4  "accel_z"
  Frame Transfer/2(Out2) -> Bus Creator/3  "accel_y"
  Frame Transfer/1(Out1) -> Bus Creator/2  "accel_x"
  Bus Selector/4 -> Frame Transfer/3(In3)  "<accel_z>"
  Bus Selector/3 -> Frame Transfer/2(In2)  "<accel_y>"
  Bus Selector/2 -> Frame Transfer/1(In1)  "<accel_x>"
  In1/1 -> Bus Selector/1
  Bus Creator/1 -> Out1/1
  Bus Selector/1 -> Bus Creator/1  "<time>"
  Bus Selector/8 -> Bus Creator/8  "<nChange>"

== system TESTENV_NAVI/FlightControl/TEST_Filter/sensor data frame transfer/SensorFrame to BodyFrame2 ==
  In1 : Inport
  Bus Creator : BusCreator  Inputs=8
  Bus Selector : BusSelector  OutputSignals=time,accel_x,accel_y,accel_z,gyro_x,gyro_y,gyro_z,nChange
  Frame Transfer : Subsystem
  Frame Transfer1 : Subsystem
  Out1 : Outport
  wires:
  Bus Selector/1 -> Bus Creator/1  "<time>"
  Bus Creator/1 -> Out1/1
  In1/1 -> Bus Selector/1
  Bus Selector/2 -> Frame Transfer/1(In1)  "<accel_x>"
  Bus Selector/3 -> Frame Transfer/2(In2)  "<accel_y>"
  Bus Selector/4 -> Frame Transfer/3(In3)  "<accel_z>"
  Frame Transfer/1(Out1) -> Bus Creator/2  "accel_x"
  Frame Transfer/2(Out2) -> Bus Creator/3  "accel_y"
  Frame Transfer/3(Out3) -> Bus Creator/4  "accel_z"
  Bus Selector/5 -> Frame Transfer1/1(In1)  "<gyro_x>"
  Bus Selector/6 -> Frame Transfer1/2(In2)  "<gyro_y>"
  Bus Selector/7 -> Frame Transfer1/3(In3)  "<gyro_z>"
  Frame Transfer1/1(Out1) -> Bus Creator/5  "gyro_x"
  Frame Transfer1/2(Out2) -> Bus Creator/6  "gyro_y"
  Frame Transfer1/3(Out3) -> Bus Creator/7  "gyro_z"
  Bus Selector/8 -> Bus Creator/8  "<nChange>"

== system TESTENV_NAVI/FlightControl/TEST_Filter/sensor data frame transfer/SensorFrame to BodyFrame3 ==
  In1 : Inport
  Bus Creator : BusCreator  Inputs=5
  Bus Selector : BusSelector  OutputSignals=time,mag_x,mag_y,mag_z,nChange
  Frame Transfer : Subsystem
  Out1 : Outport
  wires:
  Frame Transfer/3(Out3) -> Bus Creator/4  "mag_z"
  Frame Transfer/2(Out2) -> Bus Creator/3  "mag_y"
  Frame Transfer/1(Out1) -> Bus Creator/2  "mag_x"
  Bus Selector/4 -> Frame Transfer/3(In3)  "<mag_z>"
  Bus Selector/3 -> Frame Transfer/2(In2)  "<mag_y>"
  Bus Selector/2 -> Frame Transfer/1(In1)  "<mag_x>"
  In1/1 -> Bus Selector/1
  Bus Creator/1 -> Out1/1
  Bus Selector/1 -> Bus Creator/1  "<time>"
  Bus Selector/5 -> Bus Creator/5  "<nChange>"

== system TESTENV_NAVI/FlightControl/TEST_Filter/sensor data frame transfer/SensorFrame to BodyFrame4 ==
  In1 : Inport
  Bus Creator : BusCreator  Inputs=5
  Bus Selector : BusSelector  OutputSignals=time,mag_x,mag_y,mag_z,nChange
  Frame Transfer : Subsystem
  Out1 : Outport
  wires:
  Bus Selector/1 -> Bus Creator/1  "<time>"
  Bus Creator/1 -> Out1/1
  In1/1 -> Bus Selector/1
  Bus Selector/2 -> Frame Transfer/1(In1)  "<mag_x>"
  Bus Selector/3 -> Frame Transfer/2(In2)  "<mag_y>"
  Bus Selector/4 -> Frame Transfer/3(In3)  "<mag_z>"
  Frame Transfer/1(Out1) -> Bus Creator/2  "mag_x"
  Frame Transfer/2(Out2) -> Bus Creator/3  "mag_y"
  Frame Transfer/3(Out3) -> Bus Creator/4  "mag_z"
  Bus Selector/5 -> Bus Creator/5  "<nChange>"

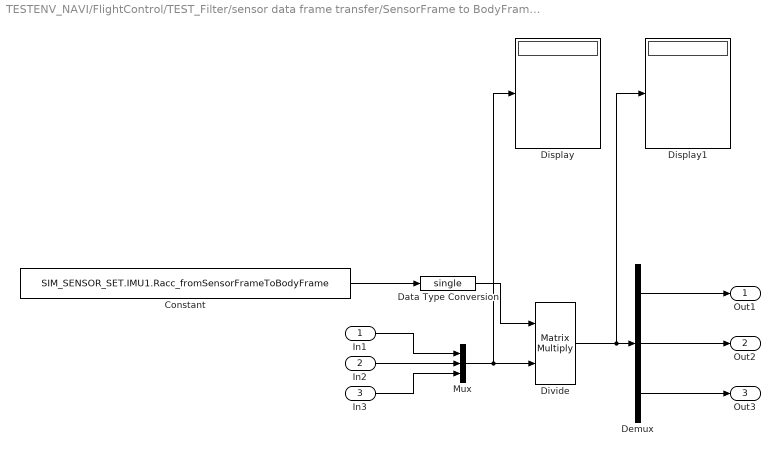
== system TESTENV_NAVI/FlightControl/TEST_Filter/sensor data frame transfer/SensorFrame to BodyFrame/Frame Transfer ==
  In1 : Inport
  In2 : Inport  Port=2
  In3 : Inport  Port=3
  Constant : Constant  Value=SIM_SENSOR_SET.IMU1.Racc_fromSensorFrameToBodyFrame
  Data Type Conversion : DataTypeConversion  OutDataTypeStr=single
  Demux : Demux  Outputs=3
  Display : Display
  Display1 : Display
  Divide : Product  Inputs=**  Multiplication=Matrix(*)
  Mux : Mux  Inputs=3
  Out1 : Outport
  Out2 : Outport  Port=2
  Out3 : Outport  Port=3
  wires:
  In2/1 -> Mux/2
  In1/1 -> Mux/1
  In3/1 -> Mux/3
  Constant/1 -> Data Type Conversion/1
  Mux/1 -> Display/1, Divide/2
  Divide/1 -> Display1/1, Demux/1
  Demux/1 -> Out1/1
  Demux/2 -> Out2/1
  Demux/3 -> Out3/1
  Data Type Conversion/1 -> Divide/1

== system TESTENV_NAVI/FlightControl/TEST_Filter/sensor data frame transfer/SensorFrame to BodyFrame/Frame Transfer1 ==
  In1 : Inport
  In2 : Inport  Port=2
  In3 : Inport  Port=3
  Constant : Constant  Value=SIM_SENSOR_SET.IMU1.Racc_fromSensorFrameToBodyFrame
  Data Type Conversion : DataTypeConversion  OutDataTypeStr=single
  Demux : Demux  Outputs=3
  Display : Display
  Display1 : Display
  Divide : Product  Inputs=**  Multiplication=Matrix(*)
  Mux : Mux  Inputs=3
  Out1 : Outport
  Out2 : Outport  Port=2
  Out3 : Outport  Port=3
  wires:
  Data Type Conversion/1 -> Divide/1
  Demux/3 -> Out3/1
  Demux/2 -> Out2/1
  Demux/1 -> Out1/1
  Divide/1 -> Demux/1, Display1/1
  Mux/1 -> Divide/2, Display/1
  Constant/1 -> Data Type Conversion/1
  In3/1 -> Mux/3
  In1/1 -> Mux/1
  In2/1 -> Mux/2

== system TESTENV_NAVI/FlightControl/TEST_Filter/sensor data frame transfer/SensorFrame to BodyFrame1/Frame Transfer ==
  In1 : Inport
  In2 : Inport  Port=2
  In3 : Inport  Port=3
  Constant : Constant  Value=SIM_SENSOR_SET.IMU1.Racc_fromSensorFrameToBodyFrame
  Data Type Conversion : DataTypeConversion  OutDataTypeStr=single
  Demux : Demux  Outputs=3
  Display : Display
  Display1 : Display
  Divide : Product  Inputs=**  Multiplication=Matrix(*)
  Mux : Mux  Inputs=3
  Out1 : Outport
  Out2 : Outport  Port=2
  Out3 : Outport  Port=3
  wires:
  Data Type Conversion/1 -> Divide/1
  Demux/3 -> Out3/1
  Demux/2 -> Out2/1
  Demux/1 -> Out1/1
  Divide/1 -> Demux/1, Display1/1
  Mux/1 -> Divide/2, Display/1
  Constant/1 -> Data Type Conversion/1
  In3/1 -> Mux/3
  In1/1 -> Mux/1
  In2/1 -> Mux/2

== system TESTENV_NAVI/FlightControl/TEST_Filter/sensor data frame transfer/SensorFrame to BodyFrame1/Frame Transfer1 ==
  In1 : Inport
  In2 : Inport  Port=2
  In3 : Inport  Port=3
  Constant : Constant  Value=SIM_SENSOR_SET.IMU1.Racc_fromSensorFrameToBodyFrame
  Data Type Conversion : DataTypeConversion  OutDataTypeStr=single
  Demux : Demux  Outputs=3
  Display : Display
  Display1 : Display
  Divide : Product  Inputs=**  Multiplication=Matrix(*)
  Mux : Mux  Inputs=3
  Out1 : Outport
  Out2 : Outport  Port=2
  Out3 : Outport  Port=3
  wires:
  In2/1 -> Mux/2
  In1/1 -> Mux/1
  In3/1 -> Mux/3
  Constant/1 -> Data Type Conversion/1
  Mux/1 -> Display/1, Divide/2
  Divide/1 -> Display1/1, Demux/1
  Demux/1 -> Out1/1
  Demux/2 -> Out2/1
  Demux/3 -> Out3/1
  Data Type Conversion/1 -> Divide/1

== system TESTENV_NAVI/FlightControl/TEST_Filter/sensor data frame transfer/SensorFrame to BodyFrame2/Frame Transfer ==
  In1 : Inport
  In2 : Inport  Port=2
  In3 : Inport  Port=3
  Constant : Constant  Value=SIM_SENSOR_SET.IMU1.Racc_fromSensorFrameToBodyFrame
  Data Type Conversion : DataTypeConversion  OutDataTypeStr=single
  Demux : Demux  Outputs=3
  Display : Display
  Display1 : Display
  Divide : Product  Inputs=**  Multiplication=Matrix(*)
  Mux : Mux  Inputs=3
  Out1 : Outport
  Out2 : Outport  Port=2
  Out3 : Outport  Port=3
  wires:
  In2/1 -> Mux/2
  In1/1 -> Mux/1
  In3/1 -> Mux/3
  Constant/1 -> Data Type Conversion/1
  Mux/1 -> Display/1, Divide/2
  Divide/1 -> Display1/1, Demux/1
  Demux/1 -> Out1/1
  Demux/2 -> Out2/1
  Demux/3 -> Out3/1
  Data Type Conversion/1 -> Divide/1

== system TESTENV_NAVI/FlightControl/TEST_Filter/sensor data frame transfer/SensorFrame to BodyFrame2/Frame Transfer1 ==
  In1 : Inport
  In2 : Inport  Port=2
  In3 : Inport  Port=3
  Constant : Constant  Value=SIM_SENSOR_SET.IMU1.Racc_fromSensorFrameToBodyFrame
  Data Type Conversion : DataTypeConversion  OutDataTypeStr=single
  Demux : Demux  Outputs=3
  Display : Display
  Display1 : Display
  Divide : Product  Inputs=**  Multiplication=Matrix(*)
  Mux : Mux  Inputs=3
  Out1 : Outport
  Out2 : Outport  Port=2
  Out3 : Outport  Port=3
  wires:
  Data Type Conversion/1 -> Divide/1
  Demux/3 -> Out3/1
  Demux/2 -> Out2/1
  Demux/1 -> Out1/1
  Divide/1 -> Demux/1, Display1/1
  Mux/1 -> Divide/2, Display/1
  Constant/1 -> Data Type Conversion/1
  In3/1 -> Mux/3
  In1/1 -> Mux/1
  In2/1 -> Mux/2

== system TESTENV_NAVI/FlightControl/TEST_Filter/sensor data frame transfer/SensorFrame to BodyFrame3/Frame Transfer ==
  In1 : Inport
  In2 : Inport  Port=2
  In3 : Inport  Port=3
  Constant : Constant  Value=SIM_SENSOR_SET.Mag1.R_fromSensorFrameToBodyFrame
  Data Type Conversion : DataTypeConversion  OutDataTypeStr=single
  Demux : Demux  Outputs=3
  Display : Display
  Display1 : Display
  Divide : Product  Inputs=**  Multiplication=Matrix(*)
  Mux : Mux  Inputs=3
  Out1 : Outport
  Out2 : Outport  Port=2
  Out3 : Outport  Port=3
  wires:
  Data Type Conversion/1 -> Divide/1
  Demux/3 -> Out3/1
  Demux/2 -> Out2/1
  Demux/1 -> Out1/1
  Divide/1 -> Demux/1, Display1/1
  Mux/1 -> Divide/2, Display/1
  Constant/1 -> Data Type Conversion/1
  In3/1 -> Mux/3
  In1/1 -> Mux/1
  In2/1 -> Mux/2

== system TESTENV_NAVI/FlightControl/TEST_Filter/sensor data frame transfer/SensorFrame to BodyFrame4/Frame Transfer ==
  In1 : Inport
  In2 : Inport  Port=2
  In3 : Inport  Port=3
  Constant : Constant  Value=SIM_SENSOR_SET.Mag2.R_fromSensorFrameToBodyFrame
  Data Type Conversion : DataTypeConversion  OutDataTypeStr=single
  Demux : Demux  Outputs=3
  Display : Display
  Display1 : Display
  Divide : Product  Inputs=**  Multiplication=Matrix(*)
  Mux : Mux  Inputs=3
  Out1 : Outport
  Out2 : Outport  Port=2
  Out3 : Outport  Port=3
  wires:
  In2/1 -> Mux/2
  In1/1 -> Mux/1
  In3/1 -> Mux/3
  Constant/1 -> Data Type Conversion/1
  Mux/1 -> Display/1, Divide/2
  Divide/1 -> Display1/1, Demux/1
  Demux/1 -> Out1/1
  Demux/2 -> Out2/1
  Demux/3 -> Out3/1
  Data Type Conversion/1 -> Divide/1

== matlab function TESTENV_NAVI/Res Data/MATLAB Function ==
  data: vel input; y output
function y = fcn(vel)

y = norm(vel(1:2));

== matlab function TESTENV_NAVI/FlightControl/SensorAndNavigation1/Subsystem1/Select VisLandParam ==
  data: planeMode input Enum: ENUM_plane_mode; P output Bus: BUS_VISUALLANDING_PARAM; P_V1000 input Bus: BUS_VISUALLANDING_PARAM; P_V10 input Bus: BUS_VISUALLANDING_PARAM
function P = fcn(planeMode,P_V1000,P_V10)
switch planeMode
    case ENUM_plane_mode.V10
        P = P_V10;
    case {ENUM_plane_mode.V1000,ENUM_plane_mode.V10s}
        P = P_V1000;
    otherwise
        P = P_V1000;
end
